simulink model "test_sys"  (R2022a)
settings: Solver=FixedStepDiscrete  StartTime=0.0  StopTime=T_final  FixedStep=T_sample  RelTol=1e-3
values from neighbouring files (symbols this model uses):
  A = [0.4 -0.3 0 0.1 ... (first row only)    [Q1_experiment.m]    (also in Run_model.m = [0.921 0 0.041 0; To_Tobias.m = [0.921 0 0.041 0; test.m)
  B = [0; -1; 1.4; 0]    [Q1_experiment.m]    (also in Run_model.m = [0.017 0.001; To_Tobias.m = [0.017 0.001; test.m)
  C = [-0.7 0 -2 0.4]    [Q1_experiment.m]    (also in Run_model.m = [1 0 0 0; To_Tobias.m = [1 0 0 0; test.m = [-0.7 0 -2 0.4)
  D = 0.2    [Q1_experiment.m]    (also in Run_model.m = zeros(n_meas,n_int); To_Tobias.m = zeros(n_meas,n_int); test.m)
  x0 = zeros(n_states,1)    [Q1_experiment.m]    (also in Run_model.m = 7*eye(n_states,1); To_Tobias.m = 7*ones(n_states,1); test.m = rand(n_states,1))
settings Model: Creator=Abelb  LastModifiedBy=Abelb
settings DebuggingCC: UnconnectedInputMsg=warning  UnconnectedOutputMsg=warning  UnconnectedLineMsg=warning
settings RTWCC: DLArmComputeVersion=19.05

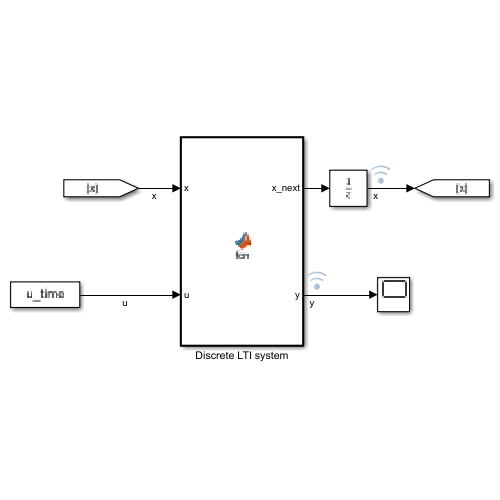
[thumbnail: Simulink's stored preview of the top-level diagram]
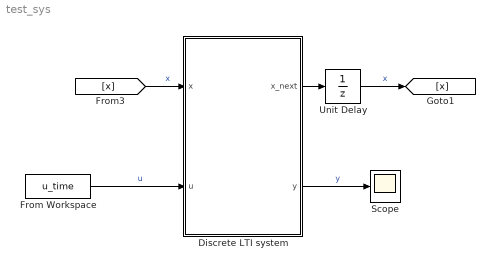
== system test_sys ==
  Discrete LTI system : MATLAB Function  TreatAsAtomicUnit=on
  From Workspace : FromWorkspace  VariableName=u_time
  Scope : Scope
  Unit Delay : UnitDelay  InitialCondition=x0  SampleTime=-1  HasFrameUpgradeWarning=on
  wires:
  Discrete LTI system/1(x_next) -> Unit Delay/1
  From Workspace/1 -> Discrete LTI system/2(u)  "u"
  Unit Delay/1 -> [x]  "x"
  [x] -> Discrete LTI system/1(x)  "x"
  Discrete LTI system/2(y) -> Scope/1  "y"

== matlab function test_sys/Discrete LTI system ==
  data: x input; x_next output; u input; y output; A parameter; C parameter; B parameter; D parameter
function [x_next,y] = fcn(x,u,A,C,B,D)
% Discrete state-space model for system

x_next = A*x + B*u;

y = C*x + D*u;
